simulink model "fast_fourier_transform_sim"  (R2020b)
settings: Solver=FixedStepDiscrete  StartTime=0.0  StopTime=stopTime  RelTol=1e-3
InitFcn:
  | initCallback
StopFcn:
  | stopCallback
undefined symbols (not defined in the file or in its folder): config, mp
settings Model: DataTypeOverride=Off  SimulationMode=accelerator  Creator=Ross  LastModifiedBy=conno
settings DataIOCC: ReturnWorkspaceOutputs=off
settings OptimizationCC: BlockReduction=off  ConditionallyExecuteInputs=off  DefaultParameterBehavior=Inlined
settings DebuggingCC: ReadBeforeWriteMsg=DisableAll  WriteAfterWriteMsg=DisableAll  WriteAfterReadMsg=DisableAll  AlgebraicLoopMsg=error  MultiTaskDSMMsg=none  SingleTaskRateTransMsg=error  PregeneratedLibrarySubsystemCodeDiagnostic=none  ArithmeticOperatorsInVariantConditions=warning
settings HardwareCC: ProdBitPerPointer=32  ProdBitPerSizeT=32  ProdBitPerPtrDiffT=32  ProdLargestAtomicFloat=None  ProdIntDivRoundTo=Undefined  ProdEndianess=Unspecified  ProdWordSize=32  ProdHWDeviceType=ASIC/FPGA->ASIC/FPGA  TargetBitPerPointer=64  TargetBitPerSizeT=64  TargetBitPerPtrDiffT=64  TargetLongLongMode=on  TargetIntDivRoundTo=Zero  TargetEndianess=LittleEndian  TargetWordSize=64  TargetHWDeviceType=Custom Processor->MATLAB Host Computer  ProdEqTarget=off
settings ModelReferenceCC: UpdateModelReferenceTargets=IfOutOfDate
settings SFSimCC: SFSimEcho=off  SimUseLocalCustomCode=off  CustomCodeUndefinedFunction=UseInterfaceOnly
settings RTWCC: RTWUseLocalCustomCode=off

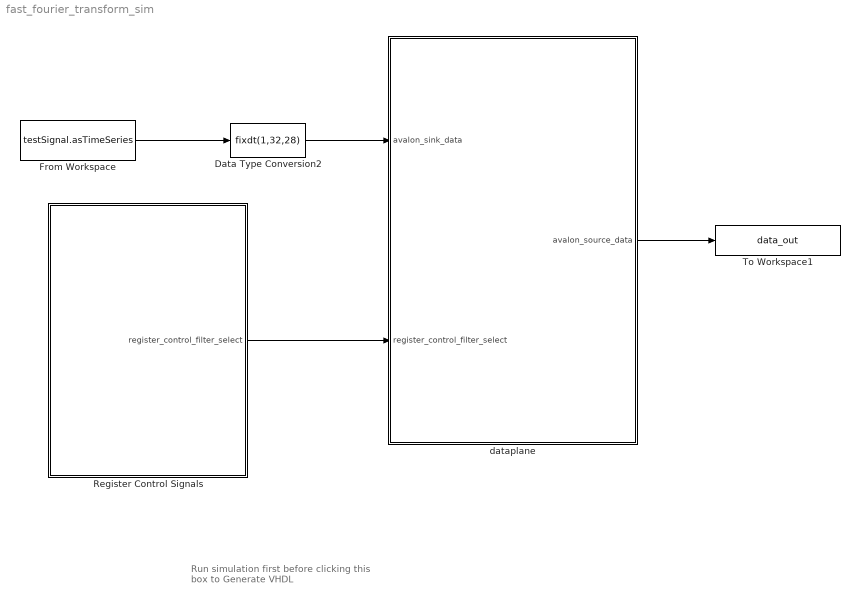
== system fast_fourier_transform_sim ==
  note: Run simulation first
      | before clicking this box to
      | Generate VHDL
  Data Type Conversion2 : DataTypeConversion  OutDataTypeStr=fixdt(1,32,28)
  From Workspace : FromWorkspace  VariableName=testSignal.asTimeSeries  SampleTime=1 / config.system.sampleClockFrequency
  Register Control Signals : Subsystem
  To Workspace1 : ToWorkspace  VariableName=data_out  SaveFormat=Timeseries  SampleTime=-1
  dataplane : Subsystem  TreatAsAtomicUnit=on
  wires:
  dataplane/1("avalon_source_data ") -> To Workspace1/1
  Register Control Signals/1(register_control_filter_select) -> dataplane/2(register_control_filter_select)
  From Workspace/1 -> Data Type Conversion2/1
  Data Type Conversion2/1 -> dataplane/1(avalon_sink_data)

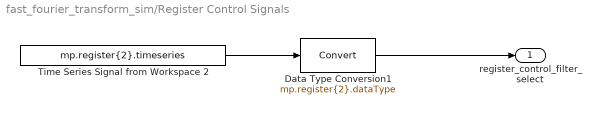
== system fast_fourier_transform_sim/Register Control Signals ==
  Data Type Conversion1 : DataTypeConversion  OutDataTypeStr=mp.register{2}.dataType  RndMeth=Nearest
  Time Series Signal from Workspace 2 : FromWorkspace  VariableName=mp.register{2}.timeseries  OutDataTypeStr=double  SampleTime=mp.Ts  OutputAfterFinalValue=Holding final value
  register_control_filter_select : Outport  VectorParamsAs1DForOutWhenUnconnected=off
  wires:
  Time Series Signal from Workspace 2/1 -> Data Type Conversion1/1
  Data Type Conversion1/1 -> register_control_filter_select/1

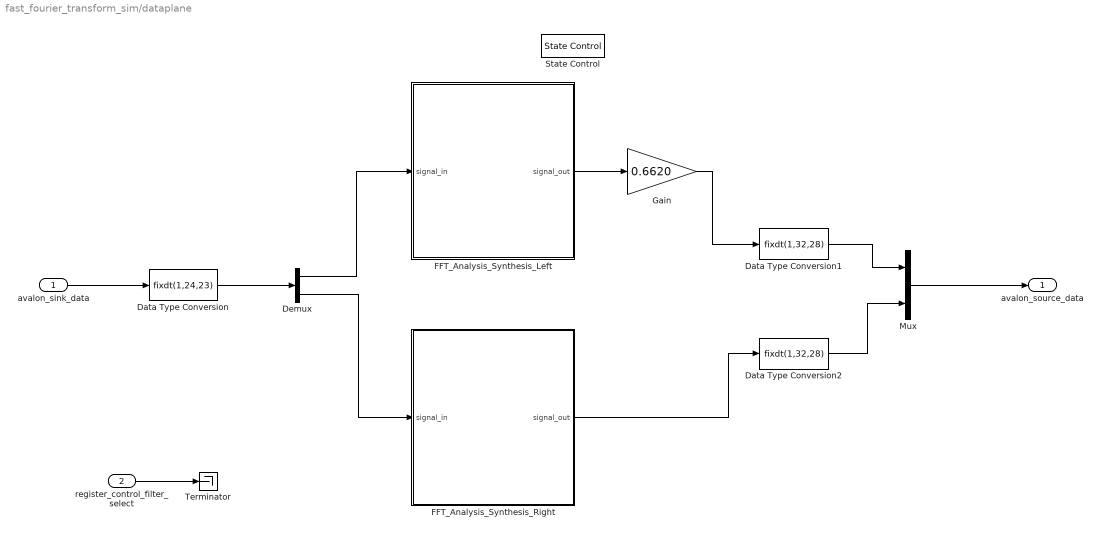
== system fast_fourier_transform_sim/dataplane ==
  avalon_sink_data : Inport
  register_control_filter_select : Inport  Port=2
  Data Type Conversion : DataTypeConversion  OutDataTypeStr=fixdt(1,24,23)
  Data Type Conversion1 : DataTypeConversion  OutDataTypeStr=fixdt(1,32,28)
  Data Type Conversion2 : DataTypeConversion  OutDataTypeStr=fixdt(1,32,28)
  Demux : Demux  Outputs=2
  FFT_Analysis_Synthesis_Left : Subsystem  TreatAsAtomicUnit=on
  FFT_Analysis_Synthesis_Right : Subsystem  TreatAsAtomicUnit=on
  Gain : Gain  Gain=0.6620
  Mux : Mux  Inputs=2
  State Control : StateControl  StateControl=Synchronous
  Terminator : Terminator
  "avalon_source_data " : Outport  InitialOutput=0  VectorParamsAs1DForOutWhenUnconnected=off
  wires:
  avalon_sink_data/1 -> Data Type Conversion/1
  Demux/1 -> FFT_Analysis_Synthesis_Left/1(signal_in)
  Data Type Conversion1/1 -> Mux/1
  Data Type Conversion2/1 -> Mux/2
  Mux/1 -> "avalon_source_data "/1
  Demux/2 -> FFT_Analysis_Synthesis_Right/1(signal_in)
  FFT_Analysis_Synthesis_Right/1(signal_out) -> Data Type Conversion2/1
  register_control_filter_select/1 -> Terminator/1
  Data Type Conversion/1 -> Demux/1
  Gain/1 -> Data Type Conversion1/1
  FFT_Analysis_Synthesis_Left/1(signal_out) -> Gain/1

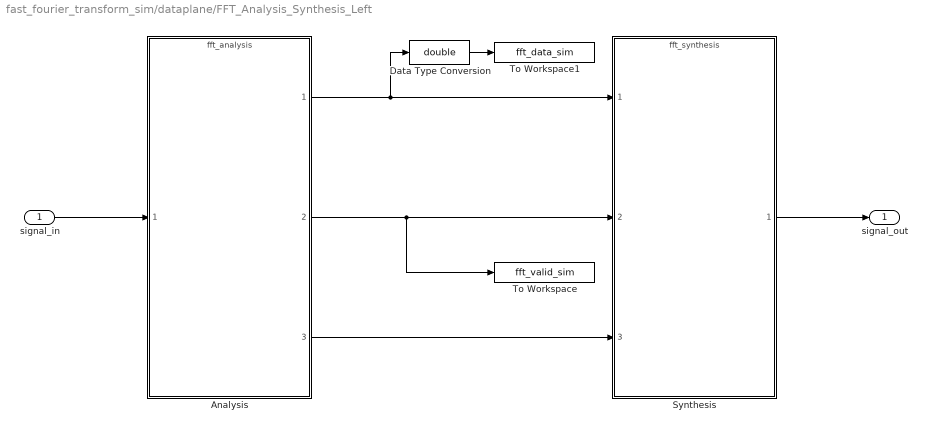
== system fast_fourier_transform_sim/dataplane/FFT_Analysis_Synthesis_Left ==
  signal_in : Inport
  Analysis : ModelReference  ModelNameDialog=fft_analysis  SimulationMode=Normal  ModelReferenceVersion=1.148
  Data Type Conversion : DataTypeConversion  OutDataTypeStr=double
  Synthesis : ModelReference  ModelNameDialog=fft_synthesis.slx  SimulationMode=Normal  ModelReferenceVersion=3.4
  To Workspace : ToWorkspace  VariableName=fft_valid_sim  SaveFormat=Timeseries  SampleTime=-1
  To Workspace1 : ToWorkspace  VariableName=fft_data_sim  SaveFormat=Timeseries  SampleTime=-1
  signal_out : Outport  VectorParamsAs1DForOutWhenUnconnected=off
  wires:
  signal_in/1 -> Analysis/1
  Synthesis/1 -> signal_out/1
  Analysis/1 -> Data Type Conversion/1, Synthesis/1
  Analysis/2 -> To Workspace/1, Synthesis/2
  Analysis/3 -> Synthesis/3
  Data Type Conversion/1 -> To Workspace1/1

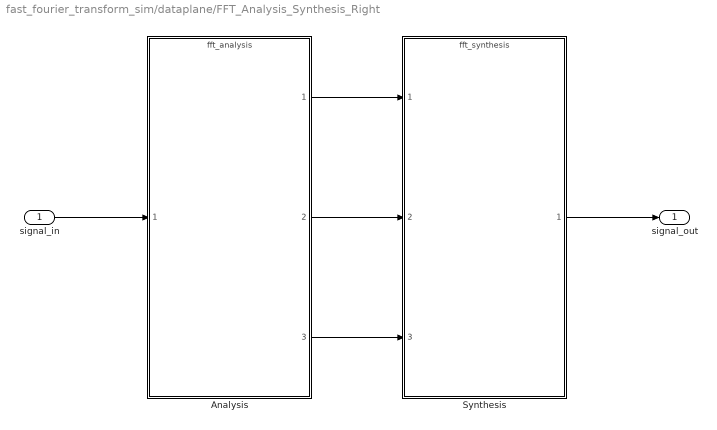
== system fast_fourier_transform_sim/dataplane/FFT_Analysis_Synthesis_Right ==
  signal_in : Inport
  Analysis : ModelReference  ModelNameDialog=fft_analysis  SimulationMode=Normal  ModelReferenceVersion=1.148
  Synthesis : ModelReference  ModelNameDialog=fft_synthesis  SimulationMode=Normal  ModelReferenceVersion=3.4
  signal_out : Outport  VectorParamsAs1DForOutWhenUnconnected=off
  wires:
  Analysis/1 -> Synthesis/1
  Analysis/3 -> Synthesis/3
  Analysis/2 -> Synthesis/2
  signal_in/1 -> Analysis/1
  Synthesis/1 -> signal_out/1
